simulink model "metareasoning"  (R2020a)
settings: Solver=FixedStepAuto  StartTime=0.0  StopTime=1000  FixedStep=0.5  RelTol=1e-3
PreLoadFcn:
  | Metareasoningpreloadfcn
InitFcn:
  | MetareasoningInitFcn
StopFcn:
  | trajectory_plot
values from neighbouring files (symbols this model uses):
  Clmax = 2.0    (= 2)    [Metareasoningpreloadfcn.m]
  Clmin = -.5    (= -0.5)    [Metareasoningpreloadfcn.m]
  g = 9.81    [Metareasoningpreloadfcn.m]
  goal_pos = [9000, 1E6, 0; -1E6, 23150+9000, 0]    [MetareasoningInitFcn.m]
  LOS_m = 9260    [Metareasoningpreloadfcn.m]
  num_ac = 2    [MetareasoningInitFcn.m]
  omega_chi = .2    (= 0.2)    [Metareasoningpreloadfcn.m]
  omega_gamma = .2    (= 0.2)    [Metareasoningpreloadfcn.m]
  omega_v = .3    (= 0.3)    [Metareasoningpreloadfcn.m]
  rho = 1.225    [Metareasoningpreloadfcn.m]
  S = 37.161    [Metareasoningpreloadfcn.m]
  tau_b = .5    (= 0.5)    [Metareasoningpreloadfcn.m]
  tau_n = .5    (= 0.5)    [Metareasoningpreloadfcn.m]
  tau_t = 1    [Metareasoningpreloadfcn.m]
  thrust_ic = 0.5*rho.*vel_ic.^2*S.*Cd    [MetareasoningInitFcn.m]
  Tmax = 25600*4.44822    (= 113874.432)    [Metareasoningpreloadfcn.m]
  W = 14515    [Metareasoningpreloadfcn.m]
undefined symbols (not defined in the file or in its folder): turnangles
libraries: asbswarm_lib x2, aerolibptmass x2, simulink x1
(part 2 of 3)

== system metareasoning/Conflict Resolution/Erzberger 2010/Cooperative Maneuvers/d_ab b right(13) ==
  States : Inport
  Turn Radius : Inport  Port=2
  Bus Selector : BusSelector  OutputSignals=Velocity,chi,x,y
  d_ab b right (13) : MATLAB Function  TreatAsAtomicUnit=on
  d_ab B Right : Outport
  wires:
  States/1 -> Bus Selector/1
  Turn Radius/1 -> d_ab b right (13)/5(R)
  Bus Selector/1 -> d_ab b right (13)/1(v)  "<Velocity>"
  Bus Selector/2 -> d_ab b right (13)/2(chi)  "<chi>"
  Bus Selector/3 -> d_ab b right (13)/3(x)  "<x>"
  d_ab b right (13)/1(d_ab) -> d_ab B Right/1
  Bus Selector/4 -> d_ab b right (13)/4(y)  "<y>"

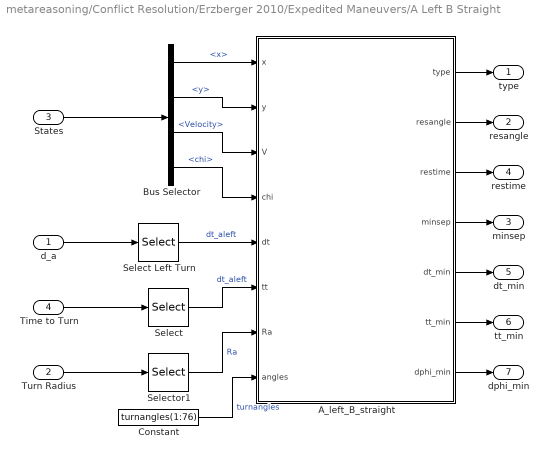
== system metareasoning/Conflict Resolution/Erzberger 2010/Expedited Maneuvers/A Left B Straight ==
  d_a : Inport
  Turn Radius : Inport  Port=2
  States : Inport  Port=3
  Time to Turn : Inport  Port=4
  A_left_B_straight : MATLAB Function  TreatAsAtomicUnit=on
  Bus Selector : BusSelector  OutputSignals=x,y,Velocity,chi
  Constant : Constant  Value=turnangles(1:76)
  "Select " : Selector  NumberOfDimensions=2  InputPortWidth=length(turnangles)  IndexOptions=Index vector (dialog),Index vector (dialog)  Indices=[1:76],1  OutputSizes=1,1
  Select Left Turn : Selector  InputPortWidth=length(turnangles)  IndexOptions=Index vector (dialog)  Indices=[1:76]  OutputSizes=1
  Selector1 : Selector  InputPortWidth=2  IndexOptions=Index vector (dialog)  Indices=[1]  OutputSizes=1
  type : Outport
  resangle : Outport  Port=2
  minsep : Outport  Port=3
  restime : Outport  Port=4
  dt_min : Outport  Port=5
  tt_min : Outport  Port=6
  dphi_min : Outport  Port=7
  wires:
  "Select "/1 -> A_left_B_straight/6(tt)  "dt_aleft"
  Bus Selector/1 -> A_left_B_straight/1(x)  "<x>"
  States/1 -> Bus Selector/1
  d_a/1 -> Select Left Turn/1
  Selector1/1 -> A_left_B_straight/7(Ra)  "Ra"
  Time to Turn/1 -> "Select "/1
  Select Left Turn/1 -> A_left_B_straight/5(dt)  "dt_aleft"
  Bus Selector/4 -> A_left_B_straight/4(chi)  "<chi>"
  Bus Selector/3 -> A_left_B_straight/3(V)  "<Velocity>"
  Constant/1 -> A_left_B_straight/8(angles)  "turnangles"
  Turn Radius/1 -> Selector1/1
  A_left_B_straight/3(restime) -> restime/1
  Bus Selector/2 -> A_left_B_straight/2(y)  "<y>"
  A_left_B_straight/1(type) -> type/1
  A_left_B_straight/5(dt_min) -> dt_min/1
  A_left_B_straight/4(minsep) -> minsep/1
  A_left_B_straight/6(tt_min) -> tt_min/1
  A_left_B_straight/7(dphi_min) -> dphi_min/1
  A_left_B_straight/2(resangle) -> resangle/1

== system metareasoning/Conflict Resolution/Erzberger 2010/Expedited Maneuvers/A Right B Straight ==
  d_a : Inport
  Turn Radius : Inport  Port=2
  States : Inport  Port=3
  Time to Turn : Inport  Port=4
  A_right_B_straight : MATLAB Function  TreatAsAtomicUnit=on
  Bus Selector : BusSelector  OutputSignals=x,y,Velocity,chi
  Constant : Constant  Value=turnangles(77:151)
  "Select " : Selector  NumberOfDimensions=2  InputPortWidth=length(turnangles)  IndexOptions=Index vector (dialog),Index vector (dialog)  Indices=[77:151],1  OutputSizes=1,1
  Select Right Turn : Selector  InputPortWidth=length(turnangles)  IndexOptions=Index vector (dialog)  Indices=[77:151]  OutputSizes=1
  Selector1 : Selector  InputPortWidth=2  IndexOptions=Index vector (dialog)  Indices=[1]  OutputSizes=1
  type : Outport
  resangle : Outport  Port=2
  minsep : Outport  Port=3
  restime : Outport  Port=4
  dt_min : Outport  Port=5
  tt_min : Outport  Port=6
  dphi_min : Outport  Port=7
  wires:
  A_right_B_straight/1(type) -> type/1
  A_right_B_straight/2(resangle) -> resangle/1
  A_right_B_straight/3(restime) -> restime/1
  A_right_B_straight/4(minsep) -> minsep/1
  Time to Turn/1 -> "Select "/1
  Bus Selector/4 -> A_right_B_straight/4(chi)  "<chi>"
  Constant/1 -> A_right_B_straight/8(angles)  "turnangles"
  Bus Selector/2 -> A_right_B_straight/2(y)  "<y>"
  Turn Radius/1 -> Selector1/1
  Select Right Turn/1 -> A_right_B_straight/5(dt)  "dt_aright"
  d_a/1 -> Select Right Turn/1
  Bus Selector/3 -> A_right_B_straight/3(V)  "<Velocity>"
  Bus Selector/1 -> A_right_B_straight/1(x)  "<x>"
  States/1 -> Bus Selector/1
  Selector1/1 -> A_right_B_straight/7(Ra)  "Ra"
  A_right_B_straight/5(dt_min) -> dt_min/1
  "Select "/1 -> A_right_B_straight/6(tt)  "dt_aright"
  A_right_B_straight/6(tt_min) -> tt_min/1
  A_right_B_straight/7(dphi_min) -> dphi_min/1

== system metareasoning/Conflict Resolution/Erzberger 2010/Expedited Maneuvers/A Straight B Left ==
  d_b : Inport
  Turn Radius : Inport  Port=2
  States : Inport  Port=3
  Time to Turn : Inport  Port=4
  Bus Selector : BusSelector  OutputSignals=x,y,Velocity,chi
  Constant : Constant  Value=turnangles(1:76)
  Find Resolution : MATLAB Function  TreatAsAtomicUnit=on
  "Select " : Selector  NumberOfDimensions=2  InputPortWidth=length(turnangles)  IndexOptions=Index vector (dialog),Index vector (dialog)  Indices=[1:76],2  OutputSizes=1,1
  Select Left Turn : Selector  InputPortWidth=length(turnangles)  IndexOptions=Index vector (dialog)  Indices=[1:76]  OutputSizes=1
  Selector1 : Selector  InputPortWidth=2  IndexOptions=Index vector (dialog)  Indices=[2]  OutputSizes=1
  type : Outport
  resangle : Outport  Port=2
  minsep : Outport  Port=3
  restime : Outport  Port=4
  dt_min : Outport  Port=5
  tt_min : Outport  Port=6
  dphi_min : Outport  Port=7
  wires:
  "Select "/1 -> Find Resolution/6(tt)  "dt_bleft"
  Bus Selector/1 -> Find Resolution/1(x)  "<x>"
  States/1 -> Bus Selector/1
  d_b/1 -> Select Left Turn/1
  Selector1/1 -> Find Resolution/7(Rb)  "Rb"
  Time to Turn/1 -> "Select "/1
  Select Left Turn/1 -> Find Resolution/5(dt)  "dt_bleft"
  Bus Selector/4 -> Find Resolution/4(chi)  "<chi>"
  Bus Selector/3 -> Find Resolution/3(V)  "<Velocity>"
  Constant/1 -> Find Resolution/8(angles)  "turnangles"
  Turn Radius/1 -> Selector1/1
  Find Resolution/3(restime) -> restime/1
  Bus Selector/2 -> Find Resolution/2(y)  "<y>"
  Find Resolution/1(type) -> type/1
  Find Resolution/5(dt_min) -> dt_min/1
  Find Resolution/4(minsep) -> minsep/1
  Find Resolution/6(tt_min) -> tt_min/1
  Find Resolution/7(dphi_min) -> dphi_min/1
  Find Resolution/2(resangle) -> resangle/1

== system metareasoning/Conflict Resolution/Erzberger 2010/Expedited Maneuvers/A Straight B Right ==
  d_b : Inport
  Turn Radius : Inport  Port=2
  States : Inport  Port=3
  Time to Turn : Inport  Port=4
  Bus Selector : BusSelector  OutputSignals=x,y,Velocity,chi
  Constant : Constant  Value=turnangles(77:151)
  Find Resolution : MATLAB Function  TreatAsAtomicUnit=on
  "Select " : Selector  NumberOfDimensions=2  InputPortWidth=length(turnangles)  IndexOptions=Index vector (dialog),Index vector (dialog)  Indices=[77:151],2  OutputSizes=1,1
  Select Right Turn : Selector  InputPortWidth=length(turnangles)  IndexOptions=Index vector (dialog)  Indices=[77:151]  OutputSizes=1
  Selector1 : Selector  InputPortWidth=2  IndexOptions=Index vector (dialog)  Indices=[2]  OutputSizes=1
  type : Outport
  resangle : Outport  Port=2
  minsep : Outport  Port=3
  restime : Outport  Port=4
  dt_min : Outport  Port=5
  tt_min : Outport  Port=6
  dphi_min : Outport  Port=7
  wires:
  "Select "/1 -> Find Resolution/6(tt)  "dt_bright"
  Bus Selector/1 -> Find Resolution/1(x)  "<x>"
  States/1 -> Bus Selector/1
  d_b/1 -> Select Right Turn/1
  Selector1/1 -> Find Resolution/7(Rb)  "Rb"
  Time to Turn/1 -> "Select "/1
  Select Right Turn/1 -> Find Resolution/5(dt)  "dt_bright"
  Bus Selector/4 -> Find Resolution/4(chi)  "<chi>"
  Bus Selector/3 -> Find Resolution/3(V)  "<Velocity>"
  Constant/1 -> Find Resolution/8(angles)  "turnangles"
  Turn Radius/1 -> Selector1/1
  Find Resolution/3(restime) -> restime/1
  Bus Selector/2 -> Find Resolution/2(y)  "<y>"
  Find Resolution/1(type) -> type/1
  Find Resolution/5(dt_min) -> dt_min/1
  Find Resolution/4(minsep) -> minsep/1
  Find Resolution/6(tt_min) -> tt_min/1
  Find Resolution/7(dphi_min) -> dphi_min/1
  Find Resolution/2(resangle) -> resangle/1

== system metareasoning/Conflict Resolution/Erzberger 2010/Expedited Maneuvers/Time To Turn ==
  Velocity : Inport
  Abs : Abs
  Constant : Constant  Value=g
  Constant1 : Constant  Value=tand(30)
  Divide : Product  Inputs=*//
  Matrix Multiply : Product  Multiplication=Matrix(*)
  Reshape : Reshape  OutputDimensionality=Row vector (2-D)
  Turn Angles : Constant  Value=turnangles  VectorParams1D=off
  Time to Turn : Outport
  wires:
  Constant1/1 -> Divide/3
  Divide/1 -> Reshape/1
  Matrix Multiply/1 -> Abs/1
  Reshape/1 -> Matrix Multiply/2
  Velocity/1 -> Divide/1
  Constant/1 -> Divide/2
  Turn Angles/1 -> Matrix Multiply/1
  Abs/1 -> Time to Turn/1

== system metareasoning/Conflict Resolution/Erzberger 2010/Expedited Maneuvers/Turn Radius (2) ==
  States : Inport
  Bus Selector : BusSelector  OutputSignals=Velocity
  Constant : Constant  Value=g*tan(deg2rad(30))
  Divide : Product  Inputs=*/
  Square : Math  Operator=square  SaturateOnIntegerOverflow=on
  Turn Radius : Outport
  wires:
  Divide/1 -> Turn Radius/1
  States/1 -> Bus Selector/1
  Constant/1 -> Divide/2
  Square/1 -> Divide/1
  Bus Selector/1 -> Square/1  "<Velocity>"

== system metareasoning/Conflict Resolution/Erzberger 2010/Expedited Maneuvers/d_a (10) ==
  States : Inport
  t : Inport  Port=2
  Turn Radius : Inport  Port=3
  Bus Selector : BusSelector  OutputSignals=Velocity,chi,x,y
  Eqn. 10 : MATLAB Function  TreatAsAtomicUnit=on
  Selector{,1..3} (4 alike) : Selector  InputPortWidth=2  IndexOptions=Index vector (dialog)  Indices=2  OutputSizes=1
  Selector4 : Selector  InputPortWidth=2  IndexOptions=Index vector (dialog)  Indices=1  OutputSizes=1
  Selector5 : Selector  NumberOfDimensions=2  InputPortWidth=3  IndexOptions=Index vector (dialog),Index vector (dialog)  Indices=1:151,1  OutputSizes=1,1
  d_a : Outport
  wires:
  Selector5/1 -> Eqn. 10/5(t)  "t"
  t/1 -> Selector5/1
  Selector4/1 -> Eqn. 10/6(Ra)  "Ra"
  Turn Radius/1 -> Selector4/1
  Selector/1 -> Eqn. 10/1(Vb)  "V_b"
  Selector1/1 -> Eqn. 10/2(hdg_b)  "hdg_b"
  Bus Selector/3 -> Selector2/1  "<x>"
  Selector3/1 -> Eqn. 10/4(y_b)  "y_b"
  Bus Selector/4 -> Selector3/1  "<y>"
  Selector2/1 -> Eqn. 10/3(x_b)  "x_b"
  Bus Selector/2 -> Selector1/1  "<chi>"
  Bus Selector/1 -> Selector/1  "<Velocity>"
  States/1 -> Bus Selector/1
  Eqn. 10/1(da) -> d_a/1

== system metareasoning/Conflict Resolution/Erzberger 2010/Expedited Maneuvers/d_b (11) ==
  States : Inport
  t : Inport  Port=2
  Turn Radius : Inport  Port=3
  Bus Selector : BusSelector  OutputSignals=Velocity,chi,x,y
  Eqn. 10 : MATLAB Function  TreatAsAtomicUnit=on
  Selector : Selector  InputPortWidth=2  IndexOptions=Index vector (dialog)  Indices=1  OutputSizes=1
  Selector{1..4} (4 alike) : Selector  InputPortWidth=2  IndexOptions=Index vector (dialog)  Indices=2  OutputSizes=1
  Selector5 : Selector  NumberOfDimensions=2  InputPortWidth=3  IndexOptions=Index vector (dialog),Index vector (dialog)  Indices=1:151,2  OutputSizes=1,1
  d_b : Outport
  wires:
  Selector5/1 -> Eqn. 10/5(t)  "t"
  t/1 -> Selector5/1
  Selector4/1 -> Eqn. 10/6(Rb)  "Rb"
  Turn Radius/1 -> Selector4/1
  Selector/1 -> Eqn. 10/1(Va)  "V_a"
  Selector1/1 -> Eqn. 10/2(hdgb)  "hdg_b"
  Bus Selector/3 -> Selector2/1  "<x>"
  Selector3/1 -> Eqn. 10/4(yb)  "y_b"
  Bus Selector/4 -> Selector3/1  "<y>"
  Selector2/1 -> Eqn. 10/3(xb)  "x_b"
  Bus Selector/2 -> Selector1/1  "<chi>"
  Bus Selector/1 -> Selector/1  "<Velocity>"
  States/1 -> Bus Selector/1
  Eqn. 10/1(db) -> d_b/1

== system metareasoning/Conflict Resolution/Erzberger 2010/Standard Maneuvers/A Left B Straight ==
  d_a : Inport
  Turn Radius : Inport  Port=2
  States : Inport  Port=3
  Time to Turn : Inport  Port=4
  A_left_B_straight : MATLAB Function  TreatAsAtomicUnit=on
  Bus Selector : BusSelector  OutputSignals=x,y,Velocity,chi
  Constant : Constant  Value=turnangles(1:76)
  "Select " : Selector  NumberOfDimensions=2  InputPortWidth=length(turnangles)  IndexOptions=Index vector (dialog),Index vector (dialog)  Indices=[1:76],1  OutputSizes=1,1
  Select Left Turn : Selector  InputPortWidth=length(turnangles)  IndexOptions=Index vector (dialog)  Indices=[1:76]  OutputSizes=1
  Selector1 : Selector  InputPortWidth=2  IndexOptions=Index vector (dialog)  Indices=[1]  OutputSizes=1
  type : Outport
  resangle : Outport  Port=2
  minsep : Outport  Port=3
  restime : Outport  Port=4
  dt_min : Outport  Port=5
  tt_min : Outport  Port=6
  dphi_min : Outport  Port=7
  wires:
  "Select "/1 -> A_left_B_straight/6(tt)  "dt_aleft"
  Bus Selector/1 -> A_left_B_straight/1(x)  "<x>"
  States/1 -> Bus Selector/1
  d_a/1 -> Select Left Turn/1
  Selector1/1 -> A_left_B_straight/7(Ra)  "Ra"
  Time to Turn/1 -> "Select "/1
  Select Left Turn/1 -> A_left_B_straight/5(dt)  "dt_aleft"
  Bus Selector/4 -> A_left_B_straight/4(chi)  "<chi>"
  Bus Selector/3 -> A_left_B_straight/3(V)  "<Velocity>"
  Constant/1 -> A_left_B_straight/8(angles)  "turnangles"
  Turn Radius/1 -> Selector1/1
  A_left_B_straight/3(restime) -> restime/1
  Bus Selector/2 -> A_left_B_straight/2(y)  "<y>"
  A_left_B_straight/1(type) -> type/1
  A_left_B_straight/5(dt_min) -> dt_min/1
  A_left_B_straight/4(minsep) -> minsep/1
  A_left_B_straight/6(tt_min) -> tt_min/1
  A_left_B_straight/7(dphi_min) -> dphi_min/1
  A_left_B_straight/2(resangle) -> resangle/1

== system metareasoning/Conflict Resolution/Erzberger 2010/Standard Maneuvers/A Right B Straight ==
  d_a : Inport
  Turn Radius : Inport  Port=2
  States : Inport  Port=3
  Time to Turn : Inport  Port=4
  A_right_B_straight : MATLAB Function  TreatAsAtomicUnit=on
  Bus Selector : BusSelector  OutputSignals=x,y,Velocity,chi
  Constant : Constant  Value=turnangles(77:151)
  "Select " : Selector  NumberOfDimensions=2  InputPortWidth=length(turnangles)  IndexOptions=Index vector (dialog),Index vector (dialog)  Indices=[77:151],1  OutputSizes=1,1
  Select Right Turn : Selector  InputPortWidth=length(turnangles)  IndexOptions=Index vector (dialog)  Indices=[77:151]  OutputSizes=1
  Selector1 : Selector  InputPortWidth=2  IndexOptions=Index vector (dialog)  Indices=[1]  OutputSizes=1
  type : Outport
  resangle : Outport  Port=2
  minsep : Outport  Port=3
  restime : Outport  Port=4
  dt_min : Outport  Port=5
  tt_min : Outport  Port=6
  dphi_min : Outport  Port=7
  wires:
  A_right_B_straight/1(type) -> type/1
  A_right_B_straight/2(resangle) -> resangle/1
  A_right_B_straight/3(restime) -> restime/1
  A_right_B_straight/4(minsep) -> minsep/1
  Time to Turn/1 -> "Select "/1
  Bus Selector/4 -> A_right_B_straight/4(chi)  "<chi>"
  Constant/1 -> A_right_B_straight/8(angles)  "turnangles"
  Bus Selector/2 -> A_right_B_straight/2(y)  "<y>"
  Turn Radius/1 -> Selector1/1
  Select Right Turn/1 -> A_right_B_straight/5(dt)  "dt_aright"
  d_a/1 -> Select Right Turn/1
  Bus Selector/3 -> A_right_B_straight/3(V)  "<Velocity>"
  Bus Selector/1 -> A_right_B_straight/1(x)  "<x>"
  States/1 -> Bus Selector/1
  Selector1/1 -> A_right_B_straight/7(Ra)  "Ra"
  A_right_B_straight/5(dt_min) -> dt_min/1
  "Select "/1 -> A_right_B_straight/6(tt)  "dt_aright"
  A_right_B_straight/6(tt_min) -> tt_min/1
  A_right_B_straight/7(dphi_min) -> dphi_min/1

== system metareasoning/Conflict Resolution/Erzberger 2010/Standard Maneuvers/A Straight B Left ==
  d_b : Inport
  Turn Radius : Inport  Port=2
  States : Inport  Port=3
  Time to Turn : Inport  Port=4
  Bus Selector : BusSelector  OutputSignals=x,y,Velocity,chi
  Constant : Constant  Value=turnangles(1:76)
  Find Resolution : MATLAB Function  TreatAsAtomicUnit=on
  "Select " : Selector  NumberOfDimensions=2  InputPortWidth=length(turnangles)  IndexOptions=Index vector (dialog),Index vector (dialog)  Indices=[1:76],2  OutputSizes=1,1
  Select Left Turn : Selector  InputPortWidth=length(turnangles)  IndexOptions=Index vector (dialog)  Indices=[1:76]  OutputSizes=1
  Selector1 : Selector  InputPortWidth=2  IndexOptions=Index vector (dialog)  Indices=[2]  OutputSizes=1
  type : Outport
  resangle : Outport  Port=2
  minsep : Outport  Port=3
  restime : Outport  Port=4
  dt_min : Outport  Port=5
  tt_min : Outport  Port=6
  dphi_min : Outport  Port=7
  wires:
  "Select "/1 -> Find Resolution/6(tt)  "dt_bleft"
  Bus Selector/1 -> Find Resolution/1(x)  "<x>"
  States/1 -> Bus Selector/1
  d_b/1 -> Select Left Turn/1
  Selector1/1 -> Find Resolution/7(Rb)  "Rb"
  Time to Turn/1 -> "Select "/1
  Select Left Turn/1 -> Find Resolution/5(dt)  "dt_bleft"
  Bus Selector/4 -> Find Resolution/4(chi)  "<chi>"
  Bus Selector/3 -> Find Resolution/3(V)  "<Velocity>"
  Constant/1 -> Find Resolution/8(angles)  "turnangles"
  Turn Radius/1 -> Selector1/1
  Find Resolution/3(restime) -> restime/1
  Bus Selector/2 -> Find Resolution/2(y)  "<y>"
  Find Resolution/1(type) -> type/1
  Find Resolution/5(dt_min) -> dt_min/1
  Find Resolution/4(minsep) -> minsep/1
  Find Resolution/6(tt_min) -> tt_min/1
  Find Resolution/7(dphi_min) -> dphi_min/1
  Find Resolution/2(resangle) -> resangle/1

== system metareasoning/Conflict Resolution/Erzberger 2010/Standard Maneuvers/A Straight B Right ==
  d_b : Inport
  Turn Radius : Inport  Port=2
  States : Inport  Port=3
  Time to Turn : Inport  Port=4
  Bus Selector : BusSelector  OutputSignals=x,y,Velocity,chi
  Constant : Constant  Value=turnangles(77:151)
  Find Resolution : MATLAB Function  TreatAsAtomicUnit=on
  "Select " : Selector  NumberOfDimensions=2  InputPortWidth=length(turnangles)  IndexOptions=Index vector (dialog),Index vector (dialog)  Indices=[77:151],2  OutputSizes=1,1
  Select Right Turn : Selector  InputPortWidth=length(turnangles)  IndexOptions=Index vector (dialog)  Indices=[77:151]  OutputSizes=1
  Selector1 : Selector  InputPortWidth=2  IndexOptions=Index vector (dialog)  Indices=[2]  OutputSizes=1
  type : Outport
  resangle : Outport  Port=2
  minsep : Outport  Port=3
  restime : Outport  Port=4
  dt_min : Outport  Port=5
  tt_min : Outport  Port=6
  dphi_min : Outport  Port=7
  wires:
  "Select "/1 -> Find Resolution/6(tt)  "dt_bright"
  Bus Selector/1 -> Find Resolution/1(x)  "<x>"
  States/1 -> Bus Selector/1
  d_b/1 -> Select Right Turn/1
  Selector1/1 -> Find Resolution/7(Rb)  "Rb"
  Time to Turn/1 -> "Select "/1
  Select Right Turn/1 -> Find Resolution/5(dt)  "dt_bright"
  Bus Selector/4 -> Find Resolution/4(chi)  "<chi>"
  Bus Selector/3 -> Find Resolution/3(V)  "<Velocity>"
  Constant/1 -> Find Resolution/8(angles)  "turnangles"
  Turn Radius/1 -> Selector1/1
  Find Resolution/3(restime) -> restime/1
  Bus Selector/2 -> Find Resolution/2(y)  "<y>"
  Find Resolution/1(type) -> type/1
  Find Resolution/5(dt_min) -> dt_min/1
  Find Resolution/4(minsep) -> minsep/1
  Find Resolution/6(tt_min) -> tt_min/1
  Find Resolution/7(dphi_min) -> dphi_min/1
  Find Resolution/2(resangle) -> resangle/1

== system metareasoning/Conflict Resolution/Erzberger 2010/Standard Maneuvers/Time To Turn ==
  Velocity : Inport
  Abs : Abs
  Constant : Constant  Value=g
  Constant1 : Constant  Value=tand(15)
  Divide : Product  Inputs=*//
  Matrix Multiply : Product  Multiplication=Matrix(*)
  Reshape : Reshape  OutputDimensionality=Row vector (2-D)
  Turn Angles : Constant  Value=turnangles  VectorParams1D=off
  Time to Turn : Outport
  wires:
  Constant1/1 -> Divide/3
  Divide/1 -> Reshape/1
  Matrix Multiply/1 -> Abs/1
  Reshape/1 -> Matrix Multiply/2
  Velocity/1 -> Divide/1
  Constant/1 -> Divide/2
  Turn Angles/1 -> Matrix Multiply/1
  Abs/1 -> Time to Turn/1

== system metareasoning/Conflict Resolution/Erzberger 2010/Standard Maneuvers/Turn Radius (2) ==
  States : Inport
  Bus Selector : BusSelector  OutputSignals=Velocity
  Constant : Constant  Value=g*tan(deg2rad(15))
  Divide : Product  Inputs=*/
  Square : Math  Operator=square  SaturateOnIntegerOverflow=on
  Turn Radius : Outport
  wires:
  Divide/1 -> Turn Radius/1
  States/1 -> Bus Selector/1
  Constant/1 -> Divide/2
  Square/1 -> Divide/1
  Bus Selector/1 -> Square/1  "<Velocity>"

== system metareasoning/Conflict Resolution/Erzberger 2010/Standard Maneuvers/d_a (10) ==
  States : Inport
  t : Inport  Port=2
  Turn Radius : Inport  Port=3
  Bus Selector : BusSelector  OutputSignals=Velocity,chi,x,y
  Eqn. 10 : MATLAB Function  TreatAsAtomicUnit=on
  Selector{,1..3} (4 alike) : Selector  InputPortWidth=2  IndexOptions=Index vector (dialog)  Indices=2  OutputSizes=1
  Selector4 : Selector  InputPortWidth=2  IndexOptions=Index vector (dialog)  Indices=1  OutputSizes=1
  Selector5 : Selector  NumberOfDimensions=2  InputPortWidth=3  IndexOptions=Index vector (dialog),Index vector (dialog)  Indices=1:151,1  OutputSizes=1,1
  d_a : Outport
  wires:
  Selector5/1 -> Eqn. 10/5(t)  "t"
  t/1 -> Selector5/1
  Selector4/1 -> Eqn. 10/6(Ra)  "Ra"
  Turn Radius/1 -> Selector4/1
  Selector/1 -> Eqn. 10/1(Vb)  "V_b"
  Selector1/1 -> Eqn. 10/2(hdg_b)  "hdg_b"
  Bus Selector/3 -> Selector2/1  "<x>"
  Selector3/1 -> Eqn. 10/4(y_b)  "y_b"
  Bus Selector/4 -> Selector3/1  "<y>"
  Selector2/1 -> Eqn. 10/3(x_b)  "x_b"
  Bus Selector/2 -> Selector1/1  "<chi>"
  Bus Selector/1 -> Selector/1  "<Velocity>"
  States/1 -> Bus Selector/1
  Eqn. 10/1(da) -> d_a/1

== system metareasoning/Conflict Resolution/Erzberger 2010/Standard Maneuvers/d_b (11) ==
  States : Inport
  t : Inport  Port=2
  Turn Radius : Inport  Port=3
  Bus Selector : BusSelector  OutputSignals=Velocity,chi,x,y
  Eqn. 10 : MATLAB Function  TreatAsAtomicUnit=on
  Selector : Selector  InputPortWidth=2  IndexOptions=Index vector (dialog)  Indices=1  OutputSizes=1
  Selector{1..4} (4 alike) : Selector  InputPortWidth=2  IndexOptions=Index vector (dialog)  Indices=2  OutputSizes=1
  Selector5 : Selector  NumberOfDimensions=2  InputPortWidth=3  IndexOptions=Index vector (dialog),Index vector (dialog)  Indices=1:151,2  OutputSizes=1,1
  d_b : Outport
  wires:
  Selector5/1 -> Eqn. 10/5(t)  "t"
  t/1 -> Selector5/1
  Selector4/1 -> Eqn. 10/6(Rb)  "Rb"
  Turn Radius/1 -> Selector4/1
  Selector/1 -> Eqn. 10/1(Va)  "V_a"
  Selector1/1 -> Eqn. 10/2(hdgb)  "hdg_b"
  Bus Selector/3 -> Selector2/1  "<x>"
  Selector3/1 -> Eqn. 10/4(yb)  "y_b"
  Bus Selector/4 -> Selector3/1  "<y>"
  Selector2/1 -> Eqn. 10/3(xb)  "x_b"
  Bus Selector/2 -> Selector1/1  "<chi>"
  Bus Selector/1 -> Selector/1  "<Velocity>"
  States/1 -> Bus Selector/1
  Eqn. 10/1(db) -> d_b/1

== system metareasoning/Conflict Resolution/Frazzoli 2005 CR/Single-Agent Planning/Check Obstruction ==
  hdg_min : Inport
  hdg_max : Inport  Port=2
  phi : Inport  Port=3
  regions touching : Inport  Port=4
  Add : Sum  Inputs=+
  Display : Display
  Display Goal Heading : Display
  Display Max Heading : Display
  Display Min Heading : Display
  Display Obstruction Bool : Display
  GreaterThan : RelationalOperator  Operator=>  OutDataTypeStr=boolean  RndMeth=Simplest
  GreaterThanOrEqual : RelationalOperator  OutDataTypeStr=boolean  RndMeth=Simplest
  In the way? : Logic  IconShape=distinctive  AllPortsSameDT=off  OutDataTypeStr=boolean
  LessThanOrEqual : RelationalOperator  Operator=<=  OutDataTypeStr=boolean  RndMeth=Simplest
  Touching? : Logic  IconShape=distinctive  AllPortsSameDT=off  OutDataTypeStr=boolean
  Zero : Constant  Value=0  OutDataTypeStr=Inherit: Inherit via back propagation
  Goal Obstructed? : Outport
  wires:
  hdg_min/1 -> GreaterThanOrEqual/2, Display Min Heading/1
  hdg_max/1 -> LessThanOrEqual/2, Display Max Heading/1
  phi/1 -> Display Goal Heading/1, GreaterThanOrEqual/1, LessThanOrEqual/1
  GreaterThanOrEqual/1 -> In the way?/1
  LessThanOrEqual/1 -> In the way?/2
  In the way?/1 -> Touching?/2
  Add/1 -> GreaterThan/1
  Zero/1 -> GreaterThan/2
  GreaterThan/1 -> Display/1, Goal Obstructed?/1
  regions touching/1 -> Touching?/1
  Touching?/1 -> Display Obstruction Bool/1, Add/1

== system metareasoning/Conflict Resolution/Frazzoli 2005 CR/Single-Agent Planning/Intruders ==
  x : Inport
  R : Inport  Port=2
  y : Inport  Port=3
  chi : Inport  Port=4
  Minus : Sum  Inputs=+-
  Product2 : Product
  Product3 : Product
  SinCos1 : Trigonometry  Operator=sincos
  Sum2 : Sum  Inputs=|++
  xc[all] : Outport
  yc[all] : Outport  Port=2
  wires:
  SinCos1/1 -> Product3/2
  x/1 -> Sum2/1
  chi/1 -> SinCos1/1
  SinCos1/2 -> Product2/2
  Minus/1 -> yc[all]/1  "yc[all]"
  y/1 -> Minus/1
  Product2/1 -> Sum2/2
  Product3/1 -> Minus/2
  Sum2/1 -> xc[all]/1  "xc[all]"
  R/1 -> Product2/1, Product3/1

== system metareasoning/Conflict Resolution/Frazzoli 2005 CR/Single-Agent Planning/Ownship ==
  x : Inport
  R : Inport  Port=2
  y : Inport  Port=3
  chi : Inport  Port=4
  Minus : Sum  Inputs=+-
  Product : Product
  Product1 : Product
  SinCos : Trigonometry  Operator=sincos
  Sum : Sum  Inputs=|++
  xc[own] : Outport
  yc[own] : Outport  Port=2
  wires:
  x/1 -> Sum/1
  chi/1 -> SinCos/1
  Product/1 -> Sum/2
  y/1 -> Minus/1
  SinCos/2 -> Product/2
  Product1/1 -> Minus/2
  R/1 -> Product1/1, Product/1
  SinCos/1 -> Product1/2
  Sum/1 -> xc[own]/1  "xc[own]"
  Minus/1 -> yc[own]/1  "yc[own]"

== system metareasoning/Fixed-Wing UAV [All]/EOM/[thrust_dot mu_dot loadfactor_dot]/Subsystem2 ==
  In1 : Inport
  Selector1 : Selector  NumberOfDimensions=2  InputPortWidth=3  IndexOptions=Index vector (dialog),Index vector (dialog)  Indices=1:num_ac,1  OutputSizes=1,1
  Selector2 : Selector  NumberOfDimensions=2  InputPortWidth=3  IndexOptions=Index vector (dialog),Index vector (dialog)  Indices=1:num_ac,2  OutputSizes=1,1
  Selector3 : Selector  NumberOfDimensions=2  InputPortWidth=3  IndexOptions=Index vector (dialog),Index vector (dialog)  Indices=1:num_ac,3  OutputSizes=1,1
  Out1 : Outport  VectorParamsAs1DForOutWhenUnconnected=off
  Out2 : Outport  Port=2  VectorParamsAs1DForOutWhenUnconnected=off
  Out3 : Outport  Port=3  VectorParamsAs1DForOutWhenUnconnected=off
  wires:
  Selector2/1 -> Out2/1
  Selector1/1 -> Out1/1
  In1/1 -> Selector3/1, Selector1/1, Selector2/1
  Selector3/1 -> Out3/1

== matlab function metareasoning/Conflict Resolution/Erzberger 2010/Standard Maneuvers/A Straight B Right/Find Resolution ==
  data: x input; type output; y input; V input; chi input; dt input; tt input; Rb input; angles input; resangle output; restime output; minsep output; dt_min output; tt_min output; dphi_min output
function [type, resangle, restime, minsep, dt_min, tt_min, dphi_min] = A_straight_B_right(x,y, V, chi, dt, tt, Rb, angles)
    
    xa0 = x(1);
    xb0 = x(2);
    ya0 = y(1);
    yb0 = y(2);
    va = V(1);
    vb = V(2);
    hdgb = chi(2);
    hdga = 0;
    LOS_m = 9260;
    
    % turn parameters
    [dt_min, idx] = min(dt);
    tt_min = tt(idx);
    dphi_min = angles(idx);
    
    % eqn.8
    xb1 = xb0 + Rb.*sign(angles).*cos(hdgb) - Rb.*sign(angles).*cos(hdgb + angles);
    yb1 = yb0 - Rb.*sign(angles).*sin(hdgb) + Rb.*sign(angles).*sin(hdgb + angles);
    
    % a straight
    xa1 = xa0;
    ya1 = ya0 + va.*tt;
    
    % eqn.17
    dx1 = xb1 - xa1;
    dy1 = yb1 - ya1;
    vrx = vb.*sin(hdgb+angles) - va.*sin(hdga);
    vry = vb.*cos(hdgb+angles) - va.*cos(hdga);
    
    % eqn.18
    vrsq = vrx.^2 + vry.^2;
    ts_min = -(dx1.*vrx + dy1.*vry)./vrsq;
    
    % eqn. 19
    foo = dx1.*vrx + dy1.*vry;
    bar1 = dx1 - vrx.*foo./vrsq;
    bar2 = dy1 - vry.*foo./vrsq;
    ds_min = sqrt(bar1.^2 + bar2.^2);
    
    % execution times
    ts_min(ts_min < 0) = 0; % set negative values = 0
    t_exec = tt + ts_min;
    
    % find resolution
    
    %fake res parameters
    type = 2;
    resangle = 0;
    restime = 0;
    minsep = 0;
    residx = 1;
    
    %[skipping weird maxima stuff]
    
    % check for type 1
    if dt_min >= LOS_m
        type = 1;
        for i = 1:length(ds_min)
            if ds_min(i) >= LOS_m
                residx = i;
                break
            end
        end
        minsep = ds_min(residx);
        resangle = angles(residx);
        restime = t_exec(residx);
        % check for 1a
        if t_exec(residx) > 1.2 * tt_min
            type = 1.1;
            minsep = dt_min;
            resangle = dphi_min;
            restime = tt_min;
        end
    end   
end

== matlab function metareasoning/Conflict Resolution/Erzberger 2010/Expedited Maneuvers/A Left B Straight/A_left_B_straight ==
  data: x input; type output; y input; V input; chi input; dt input; tt input; Ra input; angles input; resangle output; restime output; minsep output; dt_min output; tt_min output; dphi_min output
function [type, resangle, restime, minsep, dt_min, tt_min, dphi_min] = A_left_B_straight(x,y, V, chi, dt, tt, Ra, angles)
    
    xa0 = x(1);
    xb0 = x(2);
    ya0 = y(1);
    yb0 = y(2);
    va = V(1);
    vb = V(2);
    hdgb = chi(2);
    LOS_m = 9260;
    
    % eqn.6
    xa1 = Ra.*sign(angles).* (1-cos(angles));
    ya1 = Ra.*sign(angles).* sin(angles);
    
    % eqn.9
    xb1 = xb0 + tt.*vb.*sin(hdgb);
    yb1 = yb0 + tt.*vb.*cos(hdgb);
    
    % eqn.17
    dx1 = xb1 - xa1;
    dy1 = yb1 - ya1;
    vrx = vb.*sin(hdgb) - va.*sin(angles);
    vry = vb.*cos(hdgb) - va.*cos(angles);
    
    % eqn.18
    vrsq = vrx.^2 + vry.^2;
    ts_min = -(dx1.*vrx + dy1.*vry)./vrsq;
    
    % eqn. 19
    foo = dx1.*vrx + dy1.*vry;
    bar1 = dx1 - vrx.*foo./vrsq;
    bar2 = dy1 - vry.*foo./vrsq;
    ds_min = sqrt(bar1.^2 + bar2.^2);
    
    % execution times
    ts_min(ts_min < 0) = 0; % set negative values = 0
    t_exec = tt + ts_min;
    
    % turn parameters
    [dt_min, idx] = min(dt);
    tt_min = tt(idx);
    dphi_min = angles(idx);
    
    % find resolution
    %Fake res parameters
    type = 2;
    resangle = 0;
    restime = 0;
    minsep = 0;
    residx = 1;
    
    %[skipping weird maxima stuff]
    
    % check for type 1
    if dt_min >= LOS_m
        type = 1;
        for i = length(ds_min):-1:1
            if ds_min(i) >= LOS_m
                residx = i;
                break
            end
        end
        minsep = ds_min(residx);
        resangle = angles(residx);
        restime = t_exec(residx);
        % check for 1a
        if restime > 1.2 * tt_min
            type = 1.1;
            minsep = dt_min;
            resangle = dphi_min;
            restime = tt_min;
        end
    end   
end

== matlab function metareasoning/Conflict Resolution/Erzberger 2010/Expedited Maneuvers/A Right B Straight/A_right_B_straight ==
  data: x input; type output; y input; V input; chi input; dt input; tt input; Ra input; angles input; resangle output; restime output; minsep output; dt_min output; tt_min output; dphi_min output
function [type, resangle, restime, minsep, dt_min, tt_min, dphi_min] = A_right_B_straight(x,y, V, chi, dt, tt, Ra, angles)
    
    xa0 = x(1);
    xb0 = x(2);
    ya0 = y(1);
    yb0 = y(2);
    va = V(1);
    vb = V(2);
    hdgb = chi(2);
    LOS_m = 9260;
    
    % eqn.6
    xa1 = Ra.*sign(angles).* (1-cos(angles));
    ya1 = Ra.*sign(angles).* sin(angles);
    
    % eqn.9
    xb1 = xb0 + tt.*vb.*sin(hdgb);
    yb1 = yb0 + tt.*vb.*cos(hdgb);
    
    % eqn.17
    dx1 = xb1 - xa1;
    dy1 = yb1 - ya1;
    vrx = vb.*sin(hdgb) - va.*sin(angles);
    vry = vb.*cos(hdgb) - va.*cos(angles);
    
    % eqn.18
    vrsq = vrx.^2 + vry.^2;
    ts_min = -(dx1.*vrx + dy1.*vry)./vrsq;
    
    % eqn. 19
    foo = dx1.*vrx + dy1.*vry;
    bar1 = dx1 - vrx.*foo./vrsq;
    bar2 = dy1 - vry.*foo./vrsq;
    ds_min = sqrt(bar1.^2 + bar2.^2);
    
    % execution times
    ts_min(ts_min < 0) = 0; % set negative values = 0
    t_exec = tt + ts_min;
    
    % turn parameters
    [dt_min, idx] = min(dt);
    tt_min = tt(idx);
    dphi_min = angles(idx);
    
    % find resolution
    %Fake res parameters
    type = 2;
    resangle = 0;
    restime = 0;
    minsep = 0;
    residx = 1;
    
    %[skipping weird maxima stuff]
    
    % check for type 1
    if dt_min >= LOS_m
        type = 1;
        for i = 1:length(ds_min)
            if ds_min(i) >= LOS_m
                residx = i;
                break
            end
        end
        minsep = ds_min(residx);
        resangle = angles(residx);
        restime = t_exec(residx);
        % check for 1a
        if restime > 1.2 * tt_min
            type = 1.1;
            minsep = dt_min;
            resangle = dphi_min;
            restime = tt_min;
        end
    end   
end

== matlab function metareasoning/Conflict Resolution/Erzberger 2010/Expedited Maneuvers/A Straight B Left/Find Resolution ==
  data: x input; type output; y input; V input; chi input; dt input; tt input; Rb input; angles input; resangle output; restime output; minsep output; dt_min output; tt_min output; dphi_min output
function [type, resangle, restime, minsep, dt_min, tt_min, dphi_min] = A_straight_B_left(x,y, V, chi, dt, tt, Rb, angles)
    
    xa0 = x(1);
    xb0 = x(2);
    ya0 = y(1);
    yb0 = y(2);
    va = V(1);
    vb = V(2);
    hdgb = chi(2);
    hdga = chi(1);
    LOS_m = 9260;
    
    % eqn.8
    xb1 = xb0 + Rb.*sign(angles).*cos(hdgb) - Rb.*sign(angles).*cos(hdgb+angles);
    yb1 = yb0 - Rb.*sign(angles).*sin(hdgb) + Rb.*sign(angles).*sin(hdgb+angles);
    
    % a straight
    xa1 = xa0;
    ya1 = ya0 + va.*tt;
    
    % eqn.17
    dx1 = xb1 - xa1;
    dy1 = yb1 - ya1;
    vrx = vb.*sin(hdgb+angles) - va.*sin(hdga);
    vry = vb.*cos(hdgb+angles) - va.*cos(hdga);
    
    % eqn.18
    vrsq = vrx.^2 + vry.^2;
    ts_min = -(dx1.*vrx + dy1.*vry)./vrsq;
    
    % eqn. 19
    foo = dx1.*vrx + dy1.*vry;
    bar1 = dx1 - vrx.*foo./vrsq;
    bar2 = dy1 - vry.*foo./vrsq;
    ds_min = sqrt(bar1.^2 + bar2.^2);
    
    % execution times
    ts_min(ts_min < 0) = 0; % set negative values = 0
    t_exec = tt + ts_min;
    
    % turn parameters
    [dt_min, idx] = min(dt)
    tt_min = tt(idx);
    dphi_min = angles(idx);
    
    % find resolution
    
    %fake res parameters
    type = 2;
    resangle = 0;
    restime = 0;
    minsep = 0;
    residx = 1;
    
    %[skipping weird maxima stuff]
    
    % check for type 1
    if dt_min >= LOS_m
        type = 1;
        for i = length(ds_min):-1:1
            if ds_min(i) >= LOS_m
                residx = i;
                break
            end
        end
        minsep = ds_min(residx);
        resangle = angles(residx);
        restime = t_exec(residx);
        check = 1.2*tt_min;
        
        % check for 1a
        if restime > 1.2 * tt_min
            type = 1.1;
            minsep = dt_min;
            resangle = dphi_min;
            restime = tt_min;
        end
    end   
end

== matlab function metareasoning/Conflict Resolution/Erzberger 2010/Expedited Maneuvers/A Straight B Right/Find Resolution ==
  data: x input; type output; y input; V input; chi input; dt input; tt input; Rb input; angles input; resangle output; restime output; minsep output; dt_min output; tt_min output; dphi_min output
function [type, resangle, restime, minsep, dt_min, tt_min, dphi_min] = A_straight_B_right(x,y, V, chi, dt, tt, Rb, angles)
    
    xa0 = x(1);
    xb0 = x(2);
    ya0 = y(1);
    yb0 = y(2);
    va = V(1);
    vb = V(2);
    hdgb = chi(2);
    hdga = 0;
    LOS_m = 9260;
    
    % turn parameters
    [dt_min, idx] = min(dt);
    tt_min = tt(idx);
    dphi_min = angles(idx);
    
    % eqn.8
    xb1 = xb0 + Rb.*sign(angles).*cos(hdgb) - Rb.*sign(angles).*cos(hdgb + angles);
    yb1 = yb0 - Rb.*sign(angles).*sin(hdgb) + Rb.*sign(angles).*sin(hdgb + angles);
    
    % a straight
    xa1 = xa0;
    ya1 = ya0 + va.*tt;
    
    % eqn.17
    dx1 = xb1 - xa1;
    dy1 = yb1 - ya1;
    vrx = vb.*sin(hdgb+angles) - va.*sin(hdga);
    vry = vb.*cos(hdgb+angles) - va.*cos(hdga);
    
    % eqn.18
    vrsq = vrx.^2 + vry.^2;
    ts_min = -(dx1.*vrx + dy1.*vry)./vrsq;
    
    % eqn. 19
    foo = dx1.*vrx + dy1.*vry;
    bar1 = dx1 - vrx.*foo./vrsq;
    bar2 = dy1 - vry.*foo./vrsq;
    ds_min = sqrt(bar1.^2 + bar2.^2);
    
    % execution times
    ts_min(ts_min < 0) = 0; % set negative values = 0
    t_exec = tt + ts_min;
    
    % find resolution
    
    %fake res parameters
    type = 2;
    resangle = 0;
    restime = 0;
    minsep = 0;
    residx = 1;
    
    %[skipping weird maxima stuff]
    
    % check for type 1
    if dt_min >= LOS_m
        type = 1;
        for i = 1:length(ds_min)
            if ds_min(i) >= LOS_m
                residx = i;
                break
            end
        end
        minsep = ds_min(residx);
        resangle = angles(residx);
        restime = t_exec(residx);
        % check for 1a
        if restime > 1.2 * tt_min
            type = 1.1;
            minsep = dt_min;
            resangle = dphi_min;
            restime = tt_min;
        end
    end   
end

== matlab function metareasoning/Conflict Resolution/Erzberger 2010/Standard Maneuvers/d_a (10)/Eqn. 10 ==
  data: Vb input; da output; hdg_b input; x_b input; y_b input; t input; Ra input
function da = fcn(Vb, hdg_b, x_b, y_b, t, Ra)
    turnangle = [-150:2:150].';
    turnangle = deg2rad(turnangle);
    q = (x_b + t.*Vb.*sin(hdg_b) - Ra.*sign(turnangle).*(1-cos(turnangle))).^2;
    r = (y_b + t.*Vb.*cos(hdg_b) - Ra.*sign(turnangle).*sin(turnangle)).^2;
    da = sqrt(q+r);
end

== matlab function metareasoning/Conflict Resolution/Erzberger 2010/Expedited Maneuvers/d_a (10)/Eqn. 10 ==
  data: Vb input; da output; hdg_b input; x_b input; y_b input; t input; Ra input
function da = fcn(Vb, hdg_b, x_b, y_b, t, Ra)
    turnangle = [-150:2:150].';
    turnangle = deg2rad(turnangle);
    q = (x_b + t.*Vb.*sin(hdg_b) - Ra.*sign(turnangle).*(1-cos(turnangle))).^2;
    r = (y_b + t.*Vb.*cos(hdg_b) - Ra.*sign(turnangle).*sin(turnangle)).^2;
    da = sqrt(q+r);
end

== matlab function metareasoning/Conflict Resolution/Erzberger 2010/Expedited Maneuvers/d_b (11)/Eqn. 10 ==
  data: Va input; db output; hdgb input; xb input; yb input; t input; Rb input
function db = fcn(Va, hdgb, xb, yb, t, Rb)
    turnangle = [-150:2:150].';
    turnangle = deg2rad(turnangle);
    q = (xb + Rb.*sign(turnangle).*cos(hdgb) - Rb.*sign(turnangle).*cos(hdgb + turnangle)).^2;
    r = (yb - t.*Va - Rb.*sign(turnangle).*sin(hdgb) + Rb.*sign(turnangle).*sin(hdgb + turnangle)).^2;
    db = sqrt(q + r);
end

== matlab function metareasoning/Conflict Resolution/Erzberger 2010/Cooperative Maneuvers/d_ab b right(13)/d_ab b right (13) ==
  data: v input; d_ab output; chi input; x input; y input; R input
function d_ab = fcn(v,chi,x,y,R)
    xa0 = x(1);
    xb0 = x(2);
    ya0 = y(1);
    yb0 = y(2);
    hdga = chi(1);
    hdgb = chi(2);
    va = v(1);
    vb = v(2);
    ra = R(1);
    rb = R(2);
    ta_a = [-150:2:150];
    ta_a = deg2rad(ta_a);
    ta_b = abs(va./vb.*ta_a);
    
    foo = (xb0 + rb.*sign(ta_b).*cos(hdgb) - rb.*sign(ta_b)...
            .*cos(hdgb + ta_b) - ra.*sign(ta_a).*(1-cos(ta_a))).^2;
    bar = (yb0 - rb.*sign(ta_b).*sin(hdgb) + rb.*sign(ta_b)...
            .*sin(hdgb + ta_b) - ra.*sign(ta_a).*sin(ta_a)).^2;
    d_ab = sqrt(foo + bar);
end

== matlab function metareasoning/Conflict Resolution/Erzberger 2010/Cooperative Maneuvers/d_ab b left(13)/d_ab b left (13) ==
  data: v input; d_ab output; chi input; x input; y input; R input
function d_ab = fcn(v,chi,x,y,R)
    xa0 = x(1);
    xb0 = x(2);
    ya0 = y(1);
    yb0 = y(2);
    hdga = chi(1);
    hdgb = chi(2);
    va = v(1);
    vb = v(2);
    ra = R(1);
    rb = R(2);
    ta_a = [-150:2:150];
    ta_a = deg2rad(ta_a);
    ta_b = -abs(va./vb.*ta_a);
    
    foo = (xb0 + rb.*sign(ta_b).*cos(hdgb) - rb.*sign(ta_b)...
            .*cos(hdgb + ta_b) - ra.*sign(ta_a).*(1-cos(ta_a))).^2;
    bar = (yb0 - rb.*sign(ta_b).*sin(hdgb) + rb.*sign(ta_b)...
            .*sin(hdgb + ta_b) - ra.*sign(ta_a).*sin(ta_a)).^2;
    d_ab = sqrt(foo + bar);
end

== matlab function metareasoning/Conflict Resolution/Erzberger 2010/Cooperative Maneuvers/A Left B Right/Find Resolution ==
  data: x input; type output; y input; V input; chi input; dt input; tt input; R input; angles input; resangle output; restime output; minsep output; dt_min output; tt_min output; dphi_min output
function [type, resangle, restime, minsep, dt_min, tt_min, dphi_min] = A_left_B_right(x,y, V, chi, dt, tt, R, angles)
    
    xa0 = x(1);
    xb0 = x(2);
    ya0 = y(1);
    yb0 = y(2);
    va = V(1);
    vb = V(2);
    hdgb = chi(2);
    hdga = chi(1);
    Ra = R(1);
    Rb = R(2);
    taa = angles;
    tab = abs(va./vb./angles);
    LOS_m = 9260;
    
    % turn parameters
    [dt_min, idx] = min(dt);
    tt_min = tt(idx);
    dphi_min = angles(idx);
    
    % eqn.6
    xa1 = Ra.*sign(taa).* (1-cos(taa));
    ya1 = Ra.*sign(taa).* sin(taa);
    
    % eqn.8
    xb1 = xb0 + Rb.*sign(tab).*cos(hdgb) - Rb.*sign(tab).*cos(hdgb + angles);
    yb1 = yb0 - Rb.*sign(tab).*sin(hdgb) + Rb.*sign(tab).*sin(hdgb + angles);
    
    % eqn.17
    dx1 = xb1 - xa1;
    dy1 = yb1 - ya1;
    vrx = vb.*sin(hdgb+tab) - va.*sin(hdga+taa);
    vry = vb.*cos(hdgb+tab) - va.*cos(hdga+taa);
    
    % eqn.18
    vrsq = vrx.^2 + vry.^2;
    ts_min = -(dx1.*vrx + dy1.*vry)./vrsq;
    
    % eqn. 19
    foo = dx1.*vrx + dy1.*vry;
    bar1 = dx1 - vrx.*foo./vrsq;
    bar2 = dy1 - vry.*foo./vrsq;
    ds_min = sqrt(bar1.^2 + bar2.^2);
    
    % execution times
    ts_min(ts_min < 0) = 0; % set negative values = 0
    t_exec = tt + ts_min;
    
    % find resolution
    
    %fake res parameters
    type = 2;
    resangle = 0;
    restime = 0;
    minsep = 0;
    residx = 1;
    
    %[skipping weird maxima stuff]
    
    % check for type 1
    if dt_min >= LOS_m
        type = 1;
        for i = length(ds_min):-1:1
            if ds_min(i) >= LOS_m
                residx = i;
                break
            end
        end
        minsep = ds_min(residx);
        resangle = angles(residx);
        restime = t_exec(residx);
        % check for 1a
        if restime > 1.2 * tt_min
            type = 1.1;
            minsep = dt_min;
            resangle = dphi_min;
            restime = tt_min;
        end
    end   
end

== matlab function metareasoning/Conflict Resolution/Erzberger 2010/Cooperative Maneuvers/A Right B Right/Find Resolution ==
  data: x input; type output; y input; V input; chi input; dt input; tt input; R input; angles input; resangle output; restime output; minsep output; dt_min output; tt_min output; dphi_min output
function [type, resangle, restime, minsep, dt_min, tt_min, dphi_min] = A_right_B_right(x,y, V, chi, dt, tt, R, angles)
    
    xa0 = x(1);
    xb0 = x(2);
    ya0 = y(1);
    yb0 = y(2);
    va = V(1);
    vb = V(2);
    hdgb = chi(2);
    hdga = chi(1);
    Ra = R(1);
    Rb = R(2);
    taa = angles;
    tab = abs(va./vb./angles);
    LOS_m = 9260;
    
    % turn parameters
    [dt_min, idx] = min(dt);
    tt_min = tt(idx);
    dphi_min = angles(idx);
    
    % eqn.6
    xa1 = Ra.*sign(taa).* (1-cos(taa));
    ya1 = Ra.*sign(taa).* sin(taa);
    
    % eqn.8
    xb1 = xb0 + Rb.*sign(tab).*cos(hdgb) - Rb.*sign(tab).*cos(hdgb + angles);
    yb1 = yb0 - Rb.*sign(tab).*sin(hdgb) + Rb.*sign(tab).*sin(hdgb + angles);
    
    % eqn.17
    dx1 = xb1 - xa1;
    dy1 = yb1 - ya1;
    vrx = vb.*sin(hdgb+tab) - va.*sin(hdga+taa);
    vry = vb.*cos(hdgb+tab) - va.*cos(hdga+taa);
    
    % eqn.18
    vrsq = vrx.^2 + vry.^2;
    ts_min = -(dx1.*vrx + dy1.*vry)./vrsq;
    
    % eqn. 19
    foo = dx1.*vrx + dy1.*vry;
    bar1 = dx1 - vrx.*foo./vrsq;
    bar2 = dy1 - vry.*foo./vrsq;
    ds_min = sqrt(bar1.^2 + bar2.^2);
    
    % execution times
    ts_min(ts_min < 0) = 0; % set negative values = 0
    t_exec = tt + ts_min;
    
    % find resolution
    
    %fake res parameters
    type = 2;
    resangle = 0;
    restime = 0;
    minsep = 0;
    residx = 1;
    
    %[skipping weird maxima stuff]
    
    % check for type 1
    if dt_min >= LOS_m
        type = 1;
        for i = 1:length(ds_min)
            if ds_min(i) >= LOS_m
                residx = i;
                break
            end
        end
        minsep = ds_min(residx);
        resangle = angles(residx);
        restime = t_exec(residx);
        % check for 1a
        if restime > 1.2 * tt_min
            type = 1.1;
            minsep = dt_min;
            resangle = dphi_min;
            restime = tt_min;
        end
    end   
end

== matlab function metareasoning/Conflict Resolution/Erzberger 2010/Cooperative Maneuvers/A Left B Left/Find Resolution ==
  data: x input; type output; y input; V input; chi input; dt input; tt input; R input; angles input; resangle output; restime output; minsep output; dt_min output; tt_min output; dphi_min output
function [type, resangle, restime, minsep, dt_min, tt_min, dphi_min] = A_left_B_left(x,y, V, chi, dt, tt, R, angles)
    
    xa0 = x(1);
    xb0 = x(2);
    ya0 = y(1);
    yb0 = y(2);
    va = V(1);
    vb = V(2);
    hdgb = chi(2);
    hdga = chi(1);
    Ra = R(1);
    Rb = R(2);
    taa = angles;
    tab = -abs(va./vb./angles);
    LOS_m = 9260;
    
    % turn parameters
    [dt_min, idx] = min(dt);
    tt_min = tt(idx);
    dphi_min = angles(idx);
    
    % eqn.6
    xa1 = Ra.*sign(taa).* (1-cos(taa));
    ya1 = Ra.*sign(taa).* sin(taa);
    
    % eqn.8
    xb1 = xb0 + Rb.*sign(tab).*cos(hdgb) - Rb.*sign(tab).*cos(hdgb + angles);
    yb1 = yb0 - Rb.*sign(tab).*sin(hdgb) + Rb.*sign(tab).*sin(hdgb + angles);
    
    % eqn.17
    dx1 = xb1 - xa1;
    dy1 = yb1 - ya1;
    vrx = vb.*sin(hdgb+tab) - va.*sin(hdga+taa);
    vry = vb.*cos(hdgb+tab) - va.*cos(hdga+taa);
    
    % eqn.18
    vrsq = vrx.^2 + vry.^2;
    ts_min = -(dx1.*vrx + dy1.*vry)./vrsq;
    
    % eqn. 19
    foo = dx1.*vrx + dy1.*vry;
    bar1 = dx1 - vrx.*foo./vrsq;
    bar2 = dy1 - vry.*foo./vrsq;
    ds_min = sqrt(bar1.^2 + bar2.^2);
    
    % execution times
    ts_min(ts_min < 0) = 0; % set negative values = 0
    t_exec = tt + ts_min;
    
    % find resolution
    
    %fake res parameters
    type = 2;
    resangle = 0;
    restime = 0;
    minsep = 0;
    residx = 1;
    
    %[skipping weird maxima stuff]
    
    % check for type 1
    if dt_min >= LOS_m
        type = 1;
        for i = length(ds_min):-1:1
            if ds_min(i) >= LOS_m
                residx = i;
                break
            end
        end
        minsep = ds_min(residx);
        resangle = angles(residx);
        restime = t_exec(residx);
        % check for 1a
        if restime > 1.2 * tt_min
            type = 1.1;
            minsep = dt_min;
            resangle = dphi_min;
            restime = tt_min;
        end
    end   
end

== matlab function metareasoning/Conflict Resolution/Frazzoli 2005 CR/Single-Agent Planning/Find Bearing of Reserved Region to Goal ==
  data: xc input; phi output; yc input; goal_pos input; df output
function [phi, df] = bearing(xc, yc, goal_pos)
    f = goal_pos(1:2,1) - [xc;yc];
    phi = atan2(f(1,1),f(2,1))
    df = norm(f);
end
